simulink model "gm_DUALportRAMinterface_v3"  (R2024a)
settings: Solver=FixedStepDiscrete  StartTime=0.0  StopTime=20  RelTol=1e-3
undefined symbols (not defined in the file or in its folder): magnitude, Ts
libraries: hdlsllib x226, hdlmdlgenlib x102, embmathops x6, simulink x1, dsphdlxfrm2 x1
(part 2 of 6)

== system gm_DUALportRAMinterface_v3/PL/integration_block1/FIFO_system1 ==
  data_in : Inport  OutDataTypeStr=fixdt(1, 16, 14)  PortDimensions=1  SampleTime=3.00000003e-08
  enable_output : Inport  Port=2  OutDataTypeStr=boolean  PortDimensions=1  SampleTime=3.00000003e-08
  load_fifo : Inport  Port=3  OutDataTypeStr=boolean  PortDimensions=1  SampleTime=3.00000003e-08
  Add1 : Sum  OutDataTypeStr=fixdt(0,13,0)
  Chart1 : Subsystem
  Chart2 : Subsystem
  Chart3 : Subsystem
  Constant3 : Constant  OutDataTypeStr=fixdt(0,12,0)  SampleTime=Ts
  Constant4 : Constant  Value=0  OutDataTypeStr=fixdt(1,13,0)  SampleTime=Ts
  Delay : Delay  DelayLength=2048  InitialCondition=0  UseCircularBuffer=on
  Delay1 : Delay  DelayLength=1  InitialCondition=0  SampleTime=Ts
  Delay2 : Delay  DelayLength=1  InitialCondition=0  SampleTime=Ts
  Delay3 : Delay  DelayLength=1  InitialCondition=0
  HDL FIFO1 : hdlsllib/HDL RAMs/HDL FIFO  fifo_size=4096+2048+1  mode=Classic  ratio=1  push_msg=Warning  pop_msg=Warning  show_empty=off  show_full=on  show_num=off  LabelModeActiveChoice_Mode=Classic  rst_port=off
  Logical Operator : Logic  Operator=OR  IconShape=distinctive  AllPortsSameDT=off  OutDataTypeStr=boolean
  Logical Operator1 : Logic  IconShape=distinctive  AllPortsSameDT=off  OutDataTypeStr=boolean
  Logical Operator2 : Logic  IconShape=distinctive  AllPortsSameDT=off  OutDataTypeStr=boolean
  Logical Operator3 : Logic  Operator=XOR  IconShape=distinctive  AllPortsSameDT=off  OutDataTypeStr=boolean
  Logical Operator4 : Logic  IconShape=distinctive  AllPortsSameDT=off  OutDataTypeStr=boolean
  Logical Operator5 : Logic  Operator=XOR  IconShape=distinctive  AllPortsSameDT=off  OutDataTypeStr=boolean
  Logical Operator6 : Logic  Operator=XOR  IconShape=distinctive  AllPortsSameDT=off  OutDataTypeStr=boolean
  Switch1 : Switch  Criteria=u2 ~= 0  OutDataTypeStr=fixdt(0,13,0)  SaturateOnIntegerOverflow=off  InputSameDT=off
  Switch3 : Switch  Criteria=u2 ~= 0  OutDataTypeStr=fixdt(1, 16, 14)  SaturateOnIntegerOverflow=off  InputSameDT=off
  tuneback : Delay  DelayLength=2048+4096+0  InitialCondition=0  UseCircularBuffer=on
  data_out : Outport  SampleTime=3.00000003e-08
  data_valid : Outport  Port=2  SampleTime=3.00000003e-08
  reset_fft : Outport  Port=3  SampleTime=3.00000003e-08
  FIFO_full : Outport  Port=4  SampleTime=3.00000003e-08
  wires:
  data_in/1 -> Switch3/1
  load_fifo/1 -> Chart2/1(load_FIFO1)
  Chart3/1(enable_pop) -> Logical Operator1/1, Delay2/1, Logical Operator/2, HDL FIFO1/3
  Delay/1 -> Logical Operator2/2
  Delay2/1 -> Logical Operator1/2
  Delay3/1 -> Logical Operator6/2
  HDL FIFO1/1 -> data_out/1, Switch3/3
  HDL FIFO1/2 -> Logical Operator6/1, Delay3/1, Chart2/2(full)
  Logical Operator1/1 -> Logical Operator4/1, Logical Operator3/2, Logical Operator2/1, tuneback/1, Delay/1
  Logical Operator2/1 -> Logical Operator5/1, Logical Operator3/1
  Logical Operator3/1 -> reset_fft/1
  Logical Operator4/1 -> Logical Operator5/2
  Logical Operator5/1 -> data_valid/1
  Logical Operator6/1 -> FIFO_full/1
  Switch1/1 -> Chart3/1(counter), Delay1/1
  tuneback/1 -> Logical Operator4/2
  Logical Operator/1 -> HDL FIFO1/2
  Chart2/1(enable_push) -> Switch3/2, Logical Operator/1
  Switch3/1 -> HDL FIFO1/1
  Delay1/1 -> Chart1/1(counter), Add1/1
  enable_output/1 -> Chart1/2(en_out)
  Constant4/1 -> Switch1/3
  Constant3/1 -> Add1/2
  Chart1/1(enable_counter) -> Switch1/2
  Add1/1 -> Switch1/1

== system gm_DUALportRAMinterface_v3/PL/integration_block1/FIFO_system3 ==
  data_in : Inport  OutDataTypeStr=fixdt(1, 16, 14)  PortDimensions=1  SampleTime=3.00000003e-08
  enable_output : Inport  Port=2  OutDataTypeStr=boolean  PortDimensions=1  SampleTime=3.00000003e-08
  load_fifo : Inport  Port=3  OutDataTypeStr=boolean  PortDimensions=1  SampleTime=3.00000003e-08
  Add1 : Sum  OutDataTypeStr=fixdt(0,13,0)
  Chart1 : Subsystem
  Chart2 : Subsystem
  Chart3 : Subsystem
  Constant3 : Constant  OutDataTypeStr=fixdt(0,12,0)  SampleTime=Ts
  Constant4 : Constant  Value=0  OutDataTypeStr=fixdt(1,13,0)  SampleTime=Ts
  Delay1 : Delay  DelayLength=1  InitialCondition=0  SampleTime=Ts
  Delay3 : Delay  DelayLength=1  InitialCondition=0
  HDL FIFO1 : hdlsllib/HDL RAMs/HDL FIFO  fifo_size=4096+2048+1  mode=Classic  ratio=1  push_msg=Warning  pop_msg=Warning  show_empty=off  show_full=on  show_num=off  LabelModeActiveChoice_Mode=Classic  rst_port=off
  Logical Operator : Logic  Operator=OR  IconShape=distinctive  AllPortsSameDT=off  OutDataTypeStr=boolean
  Logical Operator6 : Logic  Operator=XOR  IconShape=distinctive  AllPortsSameDT=off  OutDataTypeStr=boolean
  Switch1 : Switch  Criteria=u2 ~= 0  OutDataTypeStr=fixdt(0,13,0)  SaturateOnIntegerOverflow=off  InputSameDT=off
  Switch3 : Switch  Criteria=u2 ~= 0  OutDataTypeStr=fixdt(1, 16, 14)  SaturateOnIntegerOverflow=off  InputSameDT=off
  t : Constant  Value=double(0)  OutDataTypeStr=boolean  SampleTime=3.00000003e-08
  t1 : Constant  Value=double(0)  OutDataTypeStr=boolean  SampleTime=3.00000003e-08
  data_out : Outport  SampleTime=3.00000003e-08
  data_valid : Outport  Port=2  SampleTime=3.00000003e-08
  reset_fft : Outport  Port=3  SampleTime=3.00000003e-08
  FIFO_full : Outport  Port=4  SampleTime=3.00000003e-08
  wires:
  data_in/1 -> Switch3/1
  load_fifo/1 -> Chart2/1(load_FIFO1)
  Chart3/1(enable_pop) -> Logical Operator/2, HDL FIFO1/3
  Delay3/1 -> Logical Operator6/2
  HDL FIFO1/1 -> data_out/1, Switch3/3
  HDL FIFO1/2 -> Logical Operator6/1, Delay3/1, Chart2/2(full)
  t1/1 -> reset_fft/1
  t/1 -> data_valid/1
  Logical Operator6/1 -> FIFO_full/1
  Switch1/1 -> Chart3/1(counter), Delay1/1
  Logical Operator/1 -> HDL FIFO1/2
  Chart2/1(enable_push) -> Switch3/2, Logical Operator/1
  Switch3/1 -> HDL FIFO1/1
  Delay1/1 -> Chart1/1(counter), Add1/1
  enable_output/1 -> Chart1/2(en_out)
  Constant4/1 -> Switch1/3
  Constant3/1 -> Add1/2
  Chart1/1(enable_counter) -> Switch1/2
  Add1/1 -> Switch1/1

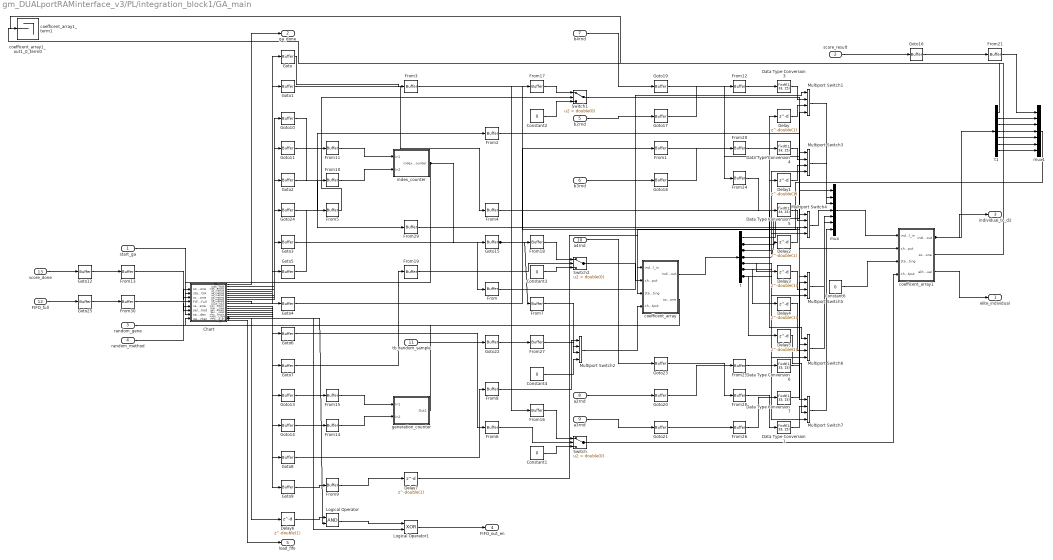
== system gm_DUALportRAMinterface_v3/PL/integration_block1/GA_main ==
  start_ga : Inport  OutDataTypeStr=boolean  PortDimensions=1  SampleTime=3.00000003e-08
  score_result : Inport  Port=2  OutDataTypeStr=fixdt(1, 33, 15)  PortDimensions=1  SampleTime=3.00000003e-08
  random_gene : Inport  Port=3  OutDataTypeStr=fixdt(0, 3, 0)  PortDimensions=1  SampleTime=3.00000003e-08
  random_method : Inport  Port=4  OutDataTypeStr=fixdt(0, 3, 0)  PortDimensions=1  SampleTime=3.00000003e-08
  b2rnd : Inport  Port=5  OutDataTypeStr=fixdt(1, 18, 15)  PortDimensions=1  SampleTime=3.00000003e-08
  b3rnd : Inport  Port=6  OutDataTypeStr=fixdt(1, 18, 15)  PortDimensions=1  SampleTime=3.00000003e-08
  b4rnd : Inport  Port=7  OutDataTypeStr=fixdt(1, 18, 15)  PortDimensions=1  SampleTime=3.00000003e-08
  a2rnd : Inport  Port=8  OutDataTypeStr=fixdt(1, 18, 15)  PortDimensions=1  SampleTime=3.00000003e-08
  a3rnd : Inport  Port=9  OutDataTypeStr=fixdt(1, 18, 15)  PortDimensions=1  SampleTime=3.00000003e-08
  a4rnd : Inport  Port=10  OutDataTypeStr=fixdt(1, 18, 15)  PortDimensions=1  SampleTime=3.00000003e-08
  tb_random_sample : Inport  Port=11  OutDataTypeStr=fixdt(0, 4, 0)  PortDimensions=1  SampleTime=3.00000003e-08
  FIFO_full : Inport  Port=12  OutDataTypeStr=boolean  PortDimensions=1  SampleTime=3.00000003e-08
  score_done : Inport  Port=13  OutDataTypeStr=boolean  PortDimensions=1  SampleTime=3.00000003e-08
  Chart : Subsystem
  Constant{1..4} (4 alike) : Constant  Value=0  OutDataTypeStr=fixdt(0, 4, 0)  SampleTime=3.00000003e-08
  Constant6 : Constant  Value=0  OutDataTypeStr=boolean  SampleTime=3.00000003e-08
  Data Type Conversion{1,3..7} (6 alike) : DataTypeConversion  OutDataTypeStr=fixdt(1, 33, 15)  SampleTime=3.00000003e-08  SaturateOnIntegerOverflow=off  RndMeth=Floor
  Delay{,1..7} (8 alike) : Delay  DelayLength=double(1)  InitialCondition=0  SampleTime=3.00000003e-08
  From{,1..21,24..30} (29 alike) : hdlmdlgenlib/Buffer
  Goto{,1..25} (26 alike) : hdlmdlgenlib/Buffer
  Logical Operator : Logic  AllPortsSameDT=off  OutDataTypeStr=boolean  SampleTime=3.00000003e-08
  Logical Operator1 : Logic  Operator=XOR  AllPortsSameDT=off  OutDataTypeStr=boolean  SampleTime=3.00000003e-08
  Multiport Switch{1,3..7} (6 alike) : MultiPortSwitch  DiagnosticForDefault=None  OutDataTypeStr=fixdt(1, 33, 15)  SampleTime=3.00000003e-08  SaturateOnIntegerOverflow=off  InputSameDT=off
  Multiport Switch2 : MultiPortSwitch  DiagnosticForDefault=None  OutDataTypeStr=fixdt(0, 4, 0)  SampleTime=3.00000003e-08  SaturateOnIntegerOverflow=off  InputSameDT=off
  Switch : Switch  Criteria=u2 > Threshold  Threshold=double(0)  OutDataTypeStr=fixdt(0, 4, 0)  SampleTime=3.00000003e-08  SaturateOnIntegerOverflow=off  InputSameDT=off
  Switch1 : Switch  Criteria=u2 > Threshold  Threshold=double(0)  OutDataTypeStr=fixdt(0, 4, 0)  SampleTime=3.00000003e-08  SaturateOnIntegerOverflow=off  InputSameDT=off
  Switch2 : Switch  Criteria=u2 > Threshold  Threshold=double(0)  OutDataTypeStr=fixdt(0, 4, 0)  SampleTime=3.00000003e-08  SaturateOnIntegerOverflow=off  InputSameDT=off
  coefficent_array : Subsystem
  coefficent_array1 : Subsystem
  coefficent_array1_out1_0_term0 : Terminator
  coefficent_array1_term1 : Terminator
  generation_counter : Subsystem
  index_counter : Subsystem
  mux : Mux  Inputs=7
  mux1 : Mux  Inputs=7
  t : Demux  Outputs=7
  t1 : Demux  Outputs=7
  elite_individual : Outport  OutDataTypeStr=fixdt(1,33,15)  SampleTime=3.00000003e-08
  ga_done : Outport  Port=2  OutDataTypeStr=boolean  SampleTime=3.00000003e-08
  individual_to_d2 : Outport  Port=3  SampleTime=3.00000003e-08
  FIFO_out_en : Outport  Port=4  SampleTime=3.00000003e-08
  load_fifo : Outport  Port=5  SampleTime=3.00000003e-08
  wires:
  score_result/1 -> Goto16/1
  b2rnd/1 -> Goto17/1
  b3rnd/1 -> Goto18/1
  b4rnd/1 -> Goto19/1
  a2rnd/1 -> Goto20/1
  a3rnd/1 -> Goto21/1
  a4rnd/1 -> Goto23/1
  tb_random_sample/1 -> Goto22/1
  FIFO_full/1 -> Goto25/1
  score_done/1 -> Goto12/1
  Chart/1(GA_done) -> ga_done/1
  Chart/17(FIFO_out_en) -> Logical Operator1/2, Logical Operator/2, Delay6/1
  Chart/18(load_fifo) -> load_fifo/1
  Delay6/1 -> Logical Operator/1
  From12/1 -> Data Type Conversion3/1
  From20/1 -> Data Type Conversion4/1
  From24/1 -> Data Type Conversion5/1
  From25/1 -> Data Type Conversion6/1
  From26/1 -> Data Type Conversion7/1
  From28/1 -> Data Type Conversion1/1
  Logical Operator/1 -> Logical Operator1/1
  Logical Operator1/1 -> FIFO_out_en/1
  coefficent_array1/1(individual_out) -> individual_to_d2/1, t1/1
  coefficent_array1/3(elite_individual) -> elite_individual/1
  Goto17/1 -> From12/1
  Goto12/1 -> From13/1
  Goto18/1 -> From20/1
  Goto16/1 -> From21/1
  Goto19/1 -> From24/1
  Goto20/1 -> From25/1
  Goto21/1 -> From26/1
  Goto22/1 -> From27/1
  Goto23/1 -> From28/1
  Goto25/1 -> From30/1
  coefficent_array1/2(sort_done) -> coefficent_array1_term1/1
  t1/1 -> coefficent_array1_out1_0_term0/1
  t1/2 -> mux1/2
  generation_counter/1(Out1) -> Chart/8(generation_counter)
  coefficent_array/1(individual_out) -> t/1
  Delay7/1 -> coefficent_array/3(start_sorting)
  index_counter/1(index_counter) -> Chart/7(sample_index), Goto15/1
  Delay/1 -> Multiport Switch1/3
  Delay1/1 -> Multiport Switch3/3
  Delay2/1 -> Multiport Switch4/3
  Delay3/1 -> Multiport Switch5/3
  Delay4/1 -> Multiport Switch6/3
  Delay5/1 -> Multiport Switch7/3
  Constant6/1 -> coefficent_array1/3(start_sorting)
  From27/1 -> Multiport Switch2/3
  Constant4/1 -> Multiport Switch2/4
  Constant3/1 -> Switch2/3
  Constant1/1 -> Switch/3
  Constant2/1 -> Switch1/3
  Data Type Conversion1/1 -> Multiport Switch7/2
  Data Type Conversion7/1 -> Multiport Switch6/2
  Data Type Conversion6/1 -> Multiport Switch5/2
  Data Type Conversion5/1 -> Multiport Switch4/2
  Data Type Conversion4/1 -> Multiport Switch3/2
  Data Type Conversion3/1 -> Multiport Switch1/2
  start_ga/1 -> Chart/2(start_GA)
  From13/1 -> Chart/3(score_done)
  From30/1 -> Chart/4(FIFO_full)
  random_gene/1 -> Chart/5(random_gene)
  random_method/1 -> Chart/6(selected_method)
  t1/3 -> mux1/3
  t1/4 -> mux1/4
  t1/5 -> mux1/5
  t1/6 -> mux1/6
  t1/7 -> mux1/7
  mux1/1 -> coefficent_array/1(individual_in)
  From21/1 -> mux1/1
  From14/1 -> generation_counter/2(In2)
  From15/1 -> generation_counter/1(In1)
  Multiport Switch2/1 -> coefficent_array/4(chose_output)
  From9/1 -> Delay7/1
  Switch2/1 -> coefficent_array/2(chose_input)
  Switch/1 -> coefficent_array1/4(chose_output)
  From10/1 -> index_counter/2(In2)
  From11/1 -> index_counter/1(In1)
  Switch1/1 -> coefficent_array1/2(chose_input)
  t/2 -> Delay/1, Multiport Switch1/4
  t/3 -> Delay1/1, Multiport Switch3/4
  t/4 -> Delay2/1, Multiport Switch4/4
  t/5 -> Delay3/1, Multiport Switch5/4
  t/6 -> Delay4/1, Multiport Switch6/4
  t/7 -> Delay5/1, Multiport Switch7/4
  mux/1 -> coefficent_array1/1(individual_in)
  coefficent_array/2(sort_done) -> Chart/1(sort_done)
  Goto14/1 -> From14/1
  Goto13/1 -> From15/1
  From7/1 -> Multiport Switch2/2
  Goto8/1 -> From8/1
  From8/1 -> Multiport Switch2/1
  Goto9/1 -> From9/1
  Goto7/1 -> From19/1
  From19/1 -> Switch2/2
  From18/1 -> Switch2/1
  Goto6/1 -> From6/1
  From6/1 -> Switch/2
  From16/1 -> Switch/1
  Goto5/1 -> From5/1
  From5/1 -> Switch1/2
  Goto10/1 -> From10/1
  Goto11/1 -> From11/1
  Goto15/1 -> From7/1, From18/1, From17/1, From16/1
  From17/1 -> Switch1/1
  Goto2/1 -> From29/1
  From29/1 -> Multiport Switch7/1
  Multiport Switch7/1 -> mux/7
  Goto1/1 -> From4/1
  From4/1 -> Multiport Switch6/1
  Multiport Switch6/1 -> mux/6
  Goto/1 -> From3/1
  From3/1 -> Multiport Switch5/1
  Multiport Switch5/1 -> mux/5
  Goto24/1 -> From2/1
  From2/1 -> Multiport Switch4/1
  Multiport Switch4/1 -> mux/4
  Goto4/1 -> From1/1
  From1/1 -> Multiport Switch3/1
  Multiport Switch3/1 -> mux/3
  Goto3/1 -> From/1
  From/1 -> Multiport Switch1/1
  Multiport Switch1/1 -> mux/2
  t/1 -> mux/1
  Chart/2(index_reset) -> Goto10/1
  Chart/3(index_increment) -> Goto11/1
  Chart/4(a2_method) -> Goto/1
  Chart/5(a3_method) -> Goto1/1
  Chart/6(a4_method) -> Goto2/1
  Chart/7(b4_method) -> Goto24/1
  Chart/8(b2_method) -> Goto3/1
  Chart/9(b3_method) -> Goto4/1
  Chart/10(slave_input) -> Goto5/1
  Chart/11(slave_output) -> Goto6/1
  Chart/12(master_input) -> Goto7/1
  Chart/13(generation_increment) -> Goto13/1
  Chart/14(generation_reset) -> Goto14/1
  Chart/15(master_output) -> Goto8/1
  Chart/16(master_sort) -> Goto9/1

== system gm_DUALportRAMinterface_v3/PL/integration_block1/Subsystem ==
  enable : Inport  OutDataTypeStr=boolean  PortDimensions=1  SampleTime=3.00000003e-08
  16bLFSR : Subsystem
  16bLFSR1 : Subsystem
  16bLFSR1_term14 : Terminator
  16bLFSR1_term15 : Terminator
  a2_random : Subsystem
  a3_random : Subsystem
  a4_random : Subsystem
  b2_random : Subsystem
  b3_random : Subsystem
  b4_random : Subsystem
  concat : hdlsllib/Logic and Bit Operations/Bit Concat  numInputs=16
  random_gene : Subsystem
  random_method : Subsystem
  random_sample : Subsystem
  random_gene_out : Outport  SampleTime=3.00000003e-08
  random_method_out : Outport  Port=2  SampleTime=3.00000003e-08
  b2_random_out : Outport  Port=3  SampleTime=3.00000003e-08
  b3_random_out : Outport  Port=4  SampleTime=3.00000003e-08
  b4_random_out : Outport  Port=5  SampleTime=3.00000003e-08
  a2_random_out : Outport  Port=6  SampleTime=3.00000003e-08
  a3_random_out : Outport  Port=7  SampleTime=3.00000003e-08
  a4_random_out : Outport  Port=8  SampleTime=3.00000003e-08
  random_sample_out : Outport  Port=9  SampleTime=3.00000003e-08
  wires:
  enable/1 -> 16bLFSR1/1(In1), 16bLFSR/1(In1)
  16bLFSR/1(y_port) -> concat/1
  16bLFSR/2(y1) -> concat/2
  16bLFSR/3(y2) -> concat/3
  16bLFSR/4(y3) -> concat/4
  16bLFSR/5(y4) -> concat/5
  16bLFSR/6(y5) -> concat/6
  16bLFSR/7(y6) -> concat/7
  16bLFSR/8(y7) -> concat/8
  16bLFSR/9(y8) -> concat/9
  16bLFSR/10(y9) -> concat/10
  16bLFSR/11(y10) -> concat/11
  16bLFSR/12(y11) -> concat/12
  16bLFSR/13(y12) -> concat/13
  16bLFSR/14(y13) -> concat/14
  16bLFSR/15(y14) -> concat/15
  16bLFSR/16(y15) -> concat/16
  16bLFSR1/1(y_port) -> a2_random/2(In2)
  16bLFSR1/2(y1) -> a3_random/2(In2)
  16bLFSR1/3(y2) -> a4_random/2(In2)
  16bLFSR1/4(y3) -> b2_random/2(In2)
  16bLFSR1/5(y4) -> b4_random/2(In2)
  16bLFSR1/6(y5) -> random_sample/1(u1)
  16bLFSR1/7(y6) -> random_sample/2(u2)
  16bLFSR1/8(y7) -> random_method/1(u1)
  16bLFSR1/9(y8) -> random_method/2(u2)
  16bLFSR1/10(y9) -> random_gene/1(u1)
  16bLFSR1/11(y10) -> random_gene/2(u2)
  16bLFSR1/12(y11) -> random_gene/3(In3)
  16bLFSR1/13(y12) -> b3_random/2(In2)
  16bLFSR1/14(y13) -> random_gene/4(In4)
  a2_random/1(Out1) -> a2_random_out/1
  a3_random/1(Out1) -> a3_random_out/1
  a4_random/1(Out1) -> a4_random_out/1
  b2_random/1(Out1) -> b2_random_out/1
  b3_random/1(Out1) -> b3_random_out/1
  b4_random/1(Out1) -> b4_random_out/1
  concat/1 -> a3_random/1(In1), a2_random/1(In1), b3_random/1(In1), b2_random/1(In1), b4_random/1(In1), a4_random/1(In1)
  random_gene/1(Out1) -> random_gene_out/1
  random_method/1(Out1) -> random_method_out/1
  random_sample/1(Out1) -> random_sample_out/1
  16bLFSR1/15(y14) -> 16bLFSR1_term14/1
  16bLFSR1/16(y15) -> 16bLFSR1_term15/1

== system gm_DUALportRAMinterface_v3/PL/integration_block1/accumulator_scorer ==
  data_in : Inport  OutDataTypeStr=fixdt(1, 28, 14)  PortDimensions=1  SampleTime=3.00000003e-08
      settings: SignalType=complex
  valid_fft : Inport  Port=2  OutDataTypeStr=boolean  PortDimensions=1  SampleTime=3.00000003e-08
  64bitmsb_finder : Subsystem
  Add : Sum  OutDataTypeStr=fixdt(1,64,32)  AccumDataTypeStr=fixdt(1,64,32)  SaturateOnIntegerOverflow=on
  Add2 : Sum  OutDataTypeStr=fixdt(1, 64, 32)  AccumDataTypeStr=fixdt(1,64,32)  SaturateOnIntegerOverflow=on
  Complex to Real-Imag : ComplexToRealImag
  Constant1 : Constant  Value=0  OutDataTypeStr=fixdt(1,26,12)  SampleTime=Ts
  Constant19 : Constant  Value=0  OutDataTypeStr=fixdt(1,26,12)  SampleTime=Ts
  Constant20 : Constant  Value=0  OutDataTypeStr=fixdt(1,64,32)  SampleTime=Ts
  Data Type Conversion : DataTypeConversion  OutDataTypeStr=fixdt(1,64,32)  SaturateOnIntegerOverflow=off  RndMeth=Floor
  Data Type Conversion1 : DataTypeConversion  OutDataTypeStr=fixdt(1,64,32)  SaturateOnIntegerOverflow=off  RndMeth=Floor
  Data Type Conversion2 : DataTypeConversion  OutDataTypeStr=fixdt(1,33,15)  SaturateOnIntegerOverflow=off  RndMeth=Floor
  Delay : Delay  DelayLength=1  InitialCondition=0  SampleTime=Ts
  Delay1 : Delay  DelayLength=63  InitialCondition=0
  Delay2 : Delay  DelayLength=1  InitialCondition=0
  Delay3 : Delay  DelayLength=4096-64  InitialCondition=0  UseCircularBuffer=on
  Logical Operator1 : Logic  IconShape=distinctive  AllPortsSameDT=off  OutDataTypeStr=boolean
  Logical Operator2 : Logic  IconShape=distinctive  AllPortsSameDT=off  OutDataTypeStr=boolean
  Magnitude Square1 : Math  Operator=magnitude^2  SignedPower=on  OutputSignalType=real  OutDataTypeStr=fixdt(1, 64, 32)  RndMeth=Zero
  Magnitude Square2 : Math  Operator=magnitude^2  SignedPower=on  OutputSignalType=real  OutDataTypeStr=fixdt(1, 64, 32)  RndMeth=Zero
  Real-Imag to Complex : RealImagToComplex
  Switch : Switch  Criteria=u2 > Threshold  OutDataTypeStr=fixdt(1, 28, 14)  SaturateOnIntegerOverflow=off  InputSameDT=off
  Switch8 : Switch  Criteria=u2 > Threshold  OutDataTypeStr=fixdt(1,64,32)  InputSameDT=off
  individual_score : Outport  SampleTime=3.00000003e-08
  individual_score_valid : Outport  Port=2  SampleTime=3.00000003e-08
  wires:
  data_in/1 -> Switch/1
  valid_fft/1 -> Logical Operator1/1, Delay3/1
  Add2/1 -> 64bitmsb_finder/1(u_port)
  Complex to Real-Imag/1 -> Data Type Conversion/1
  Complex to Real-Imag/2 -> Data Type Conversion1/1
  Constant1/1 -> Real-Imag to Complex/2
  Constant19/1 -> Real-Imag to Complex/1
  Data Type Conversion/1 -> Magnitude Square1/1
  Data Type Conversion1/1 -> Magnitude Square2/1
  Data Type Conversion2/1 -> individual_score/1
  Delay/1 -> Data Type Conversion2/1, Switch8/1
  Delay1/1 -> Logical Operator2/1
  Delay2/1 -> individual_score_valid/1
  Delay3/1 -> Logical Operator1/2
  Logical Operator1/1 -> Switch/2, Logical Operator2/2, [reset_lol], Delay1/1
  Logical Operator2/1 -> Delay2/1
  Magnitude Square1/1 -> Add2/1
  Magnitude Square2/1 -> Add2/2
  Real-Imag to Complex/1 -> Switch/3
  Switch/1 -> Complex to Real-Imag/1
  [reset_lol] -> Switch8/2
  Constant20/1 -> Switch8/3
  64bitmsb_finder/1(out1) -> Add/1
  Add/1 -> Delay/1
  Switch8/1 -> Add/2

== system gm_DUALportRAMinterface_v3/PL/integration_block1/D2/individual1 ==
  reg_in : Inport  OutDataTypeStr=fixdt(1, 33, 15)  PortDimensions=1  SampleTime=3.00000003e-08
  reg_in1 : Inport  Port=2  OutDataTypeStr=fixdt(1, 33, 15)  PortDimensions=1  SampleTime=3.00000003e-08
  reg_in2 : Inport  Port=3  OutDataTypeStr=fixdt(1, 33, 15)  PortDimensions=1  SampleTime=3.00000003e-08
  reg_in3 : Inport  Port=4  OutDataTypeStr=fixdt(1, 33, 15)  PortDimensions=1  SampleTime=3.00000003e-08
  reg_in4 : Inport  Port=5  OutDataTypeStr=fixdt(1, 33, 15)  PortDimensions=1  SampleTime=3.00000003e-08
  reg_in5 : Inport  Port=6  OutDataTypeStr=fixdt(1, 33, 15)  PortDimensions=1  SampleTime=3.00000003e-08
  reg_in6 : Inport  Port=7  OutDataTypeStr=fixdt(1, 33, 15)  PortDimensions=1  SampleTime=3.00000003e-08
  enable : Inport  Port=8  OutDataTypeStr=boolean  PortDimensions=1  SampleTime=3.00000003e-08
  Subsystem1 : Subsystem
  Subsystem2 : Subsystem
  Subsystem3 : Subsystem
  Subsystem4 : Subsystem
  Subsystem5 : Subsystem
  Subsystem6 : Subsystem
  reg_in_term0 : Terminator
  t : Constant  Value=fi(0,1,33,15)  OutDataTypeStr=fixdt(1, 33, 15)  SampleTime=3.00000003e-08
  score : Outport  SampleTime=3.00000003e-08
  a2 : Outport  Port=2  SampleTime=3.00000003e-08
  a3 : Outport  Port=3  SampleTime=3.00000003e-08
  a4 : Outport  Port=4  SampleTime=3.00000003e-08
  b2 : Outport  Port=5  SampleTime=3.00000003e-08
  b3 : Outport  Port=6  SampleTime=3.00000003e-08
  b4 : Outport  Port=7  SampleTime=3.00000003e-08
  wires:
  reg_in/1 -> reg_in_term0/1
  reg_in1/1 -> Subsystem1/1(reg_in)
  reg_in2/1 -> Subsystem2/1(reg_in)
  reg_in3/1 -> Subsystem3/1(reg_in)
  reg_in4/1 -> Subsystem4/1(reg_in)
  reg_in5/1 -> Subsystem5/1(reg_in)
  reg_in6/1 -> Subsystem6/1(reg_in)
  enable/1 -> Subsystem3/2(enable), Subsystem4/2(enable), Subsystem5/2(enable), Subsystem6/2(enable), Subsystem2/2(enable), Subsystem1/2(enable)
  t/1 -> score/1
  Subsystem1/1(reg_out) -> a2/1
  Subsystem2/1(reg_out) -> a3/1
  Subsystem3/1(reg_out) -> a4/1
  Subsystem4/1(reg_out) -> b2/1
  Subsystem5/1(reg_out) -> b3/1
  Subsystem6/1(reg_out) -> b4/1

== system gm_DUALportRAMinterface_v3/PL/integration_block1/D2/output_cast1 ==
  in : Inport  OutDataTypeStr=fixdt(1, 14, 12)  SampleTime=3.00000003e-08
  out : Outport  SampleTime=3.00000003e-08
  wires:
  in/1 -> out/1

== system gm_DUALportRAMinterface_v3/PL/integration_block1/FIFO_system1/Chart1 ==
  counter : Inport  OutDataTypeStr=fixdt(0, 13, 0)  PortDimensions=1  SampleTime=3.00000003e-08
  en_out : Inport  Port=2  OutDataTypeStr=boolean  PortDimensions=1  SampleTime=3.00000003e-08
  Chart1 : Stateflow chart  TreatAsAtomicUnit=on
      settings: PortSchema="{\"entries\":[{\"content\":{\"sides\":[{\"content\":{\"connectorIds\":[\"In2\"]},\"type\":\"ConnectorPlacement.EquallySpacedRectSide\",\"uuid\":\"9d6f18ef-7bce-40b0-94a2-758e33355834\"},{\"content\":{\"connectorIds\":[\"Out1\"],\"side\":\"RIGHT\"},\"type\":\"ConnectorPlacement.EquallySpacedRectSide\",\"uuid\":\"7bab70ba-8111-4145-9c29-33f98ce79820\"},{\"content\":{\"side\":\"TOP\"},\"type\":\"ConnectorPlacement.EquallySpacedRectSide\",\"uuid\":\"d3288235-814f-4c71-bec2-04d07c53d63c\"},{\"content\":{\"connectorIds\":[\"In1\"],\"side\":\"BOTTOM\"},\"type\":\"ConnectorPlacement.EquallySpacedRectSide\",\"uuid\":\"018953e5-55f4-4114-8f5d-132f3f7565f7\"}]},\"type\":\"ConnectorPlacement.EquallySpacedConnector\",\"uuid\":\"70011da9-c6ae-4e69-953f-1d8cbe8c7c12\"}],\"packageUris\":[\"http://schema.mathworks.com/mf0/Connector/R2020b\"],\"version\":\"1.0\"}"
  enable_counter : Outport  SampleTime=3.00000003e-08
  wires:
  Chart1/1(enable_counter) -> enable_counter/1
  en_out/1 -> Chart1/2(en_out)
  counter/1 -> Chart1/1(counter)

== system gm_DUALportRAMinterface_v3/PL/integration_block1/FIFO_system1/Chart2 ==
  load_FIFO1 : Inport  OutDataTypeStr=boolean  PortDimensions=1  SampleTime=3.00000003e-08
  full : Inport  Port=2  OutDataTypeStr=boolean  PortDimensions=1  SampleTime=3.00000003e-08
  Chart2 : Stateflow chart  TreatAsAtomicUnit=on
      settings: PortSchema="{\"entries\":[{\"content\":{\"sides\":[{\"content\":{\"connectorIds\":[\"In1\"]},\"type\":\"ConnectorPlacement.EquallySpacedRectSide\",\"uuid\":\"9d6f18ef-7bce-40b0-94a2-758e33355834\"},{\"content\":{\"connectorIds\":[\"Out1\"],\"side\":\"RIGHT\"},\"type\":\"ConnectorPlacement.EquallySpacedRectSide\",\"uuid\":\"7bab70ba-8111-4145-9c29-33f98ce79820\"},{\"content\":{\"connectorIds\":[\"In2\"],\"side\":\"TOP\"},\"type\":\"ConnectorPlacement.EquallySpacedRectSide\",\"uuid\":\"d3288235-814f-4c71-bec2-04d07c53d63c\"}]},\"type\":\"ConnectorPlacement.EquallySpacedConnector\",\"uuid\":\"70011da9-c6ae-4e69-953f-1d8cbe8c7c12\"}],\"packageUris\":[\"http://schema.mathworks.com/mf0/Connector/R2020b\"],\"version\":\"1.0\"}"
  enable_push : Outport  SampleTime=3.00000003e-08
  wires:
  Chart2/1(enable_push) -> enable_push/1
  full/1 -> Chart2/2(full)
  load_FIFO1/1 -> Chart2/1(load_FIFO1)

== system gm_DUALportRAMinterface_v3/PL/integration_block1/FIFO_system1/Chart3 ==
  counter : Inport  OutDataTypeStr=fixdt(0, 13, 0)  PortDimensions=1  SampleTime=3.00000003e-08
  Chart3 : Stateflow chart  TreatAsAtomicUnit=on
  enable_pop : Outport  SampleTime=3.00000003e-08
  wires:
  Chart3/1(enable_pop) -> enable_pop/1
  counter/1 -> Chart3/1(counter)

== system gm_DUALportRAMinterface_v3/PL/integration_block1/FIFO_system3/Chart1 ==
  counter : Inport  OutDataTypeStr=fixdt(0, 13, 0)  PortDimensions=1  SampleTime=3.00000003e-08
  en_out : Inport  Port=2  OutDataTypeStr=boolean  PortDimensions=1  SampleTime=3.00000003e-08
  Chart1 : Stateflow chart  TreatAsAtomicUnit=on
      settings: PortSchema="{\"entries\":[{\"content\":{\"sides\":[{\"content\":{\"connectorIds\":[\"In2\"]},\"type\":\"ConnectorPlacement.EquallySpacedRectSide\",\"uuid\":\"9d6f18ef-7bce-40b0-94a2-758e33355834\"},{\"content\":{\"connectorIds\":[\"Out1\"],\"side\":\"RIGHT\"},\"type\":\"ConnectorPlacement.EquallySpacedRectSide\",\"uuid\":\"7bab70ba-8111-4145-9c29-33f98ce79820\"},{\"content\":{\"side\":\"TOP\"},\"type\":\"ConnectorPlacement.EquallySpacedRectSide\",\"uuid\":\"d3288235-814f-4c71-bec2-04d07c53d63c\"},{\"content\":{\"connectorIds\":[\"In1\"],\"side\":\"BOTTOM\"},\"type\":\"ConnectorPlacement.EquallySpacedRectSide\",\"uuid\":\"018953e5-55f4-4114-8f5d-132f3f7565f7\"}]},\"type\":\"ConnectorPlacement.EquallySpacedConnector\",\"uuid\":\"70011da9-c6ae-4e69-953f-1d8cbe8c7c12\"}],\"packageUris\":[\"http://schema.mathworks.com/mf0/Connector/R2020b\"],\"version\":\"1.0\"}"
  enable_counter : Outport  SampleTime=3.00000003e-08
  wires:
  counter/1 -> Chart1/1(counter)
  en_out/1 -> Chart1/2(en_out)
  Chart1/1(enable_counter) -> enable_counter/1

== system gm_DUALportRAMinterface_v3/PL/integration_block1/FIFO_system3/Chart2 ==
  load_FIFO1 : Inport  OutDataTypeStr=boolean  PortDimensions=1  SampleTime=3.00000003e-08
  full : Inport  Port=2  OutDataTypeStr=boolean  PortDimensions=1  SampleTime=3.00000003e-08
  Chart2 : Stateflow chart  TreatAsAtomicUnit=on
      settings: PortSchema="{\"entries\":[{\"content\":{\"sides\":[{\"content\":{\"connectorIds\":[\"In1\"]},\"type\":\"ConnectorPlacement.EquallySpacedRectSide\",\"uuid\":\"9d6f18ef-7bce-40b0-94a2-758e33355834\"},{\"content\":{\"connectorIds\":[\"Out1\"],\"side\":\"RIGHT\"},\"type\":\"ConnectorPlacement.EquallySpacedRectSide\",\"uuid\":\"7bab70ba-8111-4145-9c29-33f98ce79820\"},{\"content\":{\"connectorIds\":[\"In2\"],\"side\":\"TOP\"},\"type\":\"ConnectorPlacement.EquallySpacedRectSide\",\"uuid\":\"d3288235-814f-4c71-bec2-04d07c53d63c\"}]},\"type\":\"ConnectorPlacement.EquallySpacedConnector\",\"uuid\":\"70011da9-c6ae-4e69-953f-1d8cbe8c7c12\"}],\"packageUris\":[\"http://schema.mathworks.com/mf0/Connector/R2020b\"],\"version\":\"1.0\"}"
  enable_push : Outport  SampleTime=3.00000003e-08
  wires:
  load_FIFO1/1 -> Chart2/1(load_FIFO1)
  full/1 -> Chart2/2(full)
  Chart2/1(enable_push) -> enable_push/1

== system gm_DUALportRAMinterface_v3/PL/integration_block1/FIFO_system3/Chart3 ==
  counter : Inport  OutDataTypeStr=fixdt(0, 13, 0)  PortDimensions=1  SampleTime=3.00000003e-08
  Chart3 : Stateflow chart  TreatAsAtomicUnit=on
  enable_pop : Outport  SampleTime=3.00000003e-08
  wires:
  counter/1 -> Chart3/1(counter)
  Chart3/1(enable_pop) -> enable_pop/1

== system gm_DUALportRAMinterface_v3/PL/integration_block1/GA_main/Chart ==
  sort_done : Inport  OutDataTypeStr=boolean  PortDimensions=1  SampleTime=3.00000003e-08
  start_GA : Inport  Port=2  OutDataTypeStr=boolean  PortDimensions=1  SampleTime=3.00000003e-08
  score_done : Inport  Port=3  OutDataTypeStr=boolean  PortDimensions=1  SampleTime=3.00000003e-08
  FIFO_full : Inport  Port=4  OutDataTypeStr=boolean  PortDimensions=1  SampleTime=3.00000003e-08
  random_gene : Inport  Port=5  OutDataTypeStr=fixdt(0, 3, 0)  PortDimensions=1  SampleTime=3.00000003e-08
  selected_method : Inport  Port=6  OutDataTypeStr=fixdt(0, 3, 0)  PortDimensions=1  SampleTime=3.00000003e-08
  sample_index : Inport  Port=7  OutDataTypeStr=fixdt(0, 4, 0)  PortDimensions=1  SampleTime=3.00000003e-08
  generation_counter : Inport  Port=8  OutDataTypeStr=uint16  PortDimensions=1  SampleTime=3.00000003e-08
  Chart : Stateflow chart  TreatAsAtomicUnit=on
      settings: PortSchema="{\"entries\":[{\"content\":{\"sides\":[{\"content\":{\"connectorIds\":[\"In1\",\"In2\",\"In3\",\"In4\",\"In5\",\"In6\",\"In7\",\"In8\"]},\"type\":\"ConnectorPlacement.EquallySpacedRectSide\",\"uuid\":\"62d80992-ebbf-487b-a33b-520d46b16df9\"},{\"content\":{\"connectorIds\":[\"Out1\",\"Out4\",\"Out5\",\"Out6\",\"Out8\",\"Out9\",\"Out7\",\"Out10\",\"Out11\",\"Out12\",\"Out15\",\"Out16\",\"Out13\",\"Out14\",\"Out3\",\"Out2\",\"Out17\",\"Out18\"],\"side\":\"RIGHT\"},\"type\":\"ConnectorPlacement.EquallySpacedRectSide\",\"uuid\":\"bfd840c0-5c4c-4a80-a2e3-fe311b40edf5\"},{\"content\":{\"side\":\"TOP\"},\"type\":\"ConnectorPlacement.EquallySpacedRectSide\",\"uuid\":\"4ac6e66e-dbf9-46cb-9f74-339923e0521f\"},{\"content\":{\"side\":\"BOTTOM\"},\"type\":\"ConnectorPlacement.EquallySpacedRectSide\",\"uuid\":\"c9defcd3-49e4-4e79-8497-0d4d1ccc3a89\"}]},\"type\":\"ConnectorPlacement.EquallySpacedConnector\",\"uuid\":\"f0f6ce29-0824-409a-b95e-7d534cdcf216\"}],\"packageUris\":[\"http://schema.mathworks.com/mf0/Connector/R2020b\"],\"version\":\"1.0\"}"
  GA_done : Outport  SampleTime=3.00000003e-08
  index_reset : Outport  Port=2  SampleTime=3.00000003e-08
  index_increment : Outport  Port=3  SampleTime=3.00000003e-08
  a2_method : Outport  Port=4  SampleTime=3.00000003e-08
  a3_method : Outport  Port=5  SampleTime=3.00000003e-08
  a4_method : Outport  Port=6  SampleTime=3.00000003e-08
  b4_method : Outport  Port=7  SampleTime=3.00000003e-08
  b2_method : Outport  Port=8  SampleTime=3.00000003e-08
  b3_method : Outport  Port=9  SampleTime=3.00000003e-08
  slave_input : Outport  Port=10  SampleTime=3.00000003e-08
  slave_output : Outport  Port=11  SampleTime=3.00000003e-08
  master_input : Outport  Port=12  SampleTime=3.00000003e-08
  generation_increment : Outport  Port=13  SampleTime=3.00000003e-08
  generation_reset : Outport  Port=14  SampleTime=3.00000003e-08
  master_output : Outport  Port=15  SampleTime=3.00000003e-08
  master_sort : Outport  Port=16  SampleTime=3.00000003e-08
  FIFO_out_en : Outport  Port=17  SampleTime=3.00000003e-08
  load_fifo : Outport  Port=18  SampleTime=3.00000003e-08
  wires:
  sort_done/1 -> Chart/1(sort_done)
  start_GA/1 -> Chart/2(start_GA)
  score_done/1 -> Chart/3(score_done)
  FIFO_full/1 -> Chart/4(FIFO_full)
  random_gene/1 -> Chart/5(random_gene)
  selected_method/1 -> Chart/6(selected_method)
  sample_index/1 -> Chart/7(sample_index)
  generation_counter/1 -> Chart/8(generation_counter)
  Chart/1(GA_done) -> GA_done/1
  Chart/2(index_reset) -> index_reset/1
  Chart/3(index_increment) -> index_increment/1
  Chart/4(a2_method) -> a2_method/1
  Chart/5(a3_method) -> a3_method/1
  Chart/6(a4_method) -> a4_method/1
  Chart/7(b4_method) -> b4_method/1
  Chart/8(b2_method) -> b2_method/1
  Chart/9(b3_method) -> b3_method/1
  Chart/10(slave_input) -> slave_input/1
  Chart/11(slave_output) -> slave_output/1
  Chart/12(master_input) -> master_input/1
  Chart/13(generation_increment) -> generation_increment/1
  Chart/14(generation_reset) -> generation_reset/1
  Chart/15(master_output) -> master_output/1
  Chart/16(master_sort) -> master_sort/1
  Chart/17(FIFO_out_en) -> FIFO_out_en/1
  Chart/18(load_fifo) -> load_fifo/1

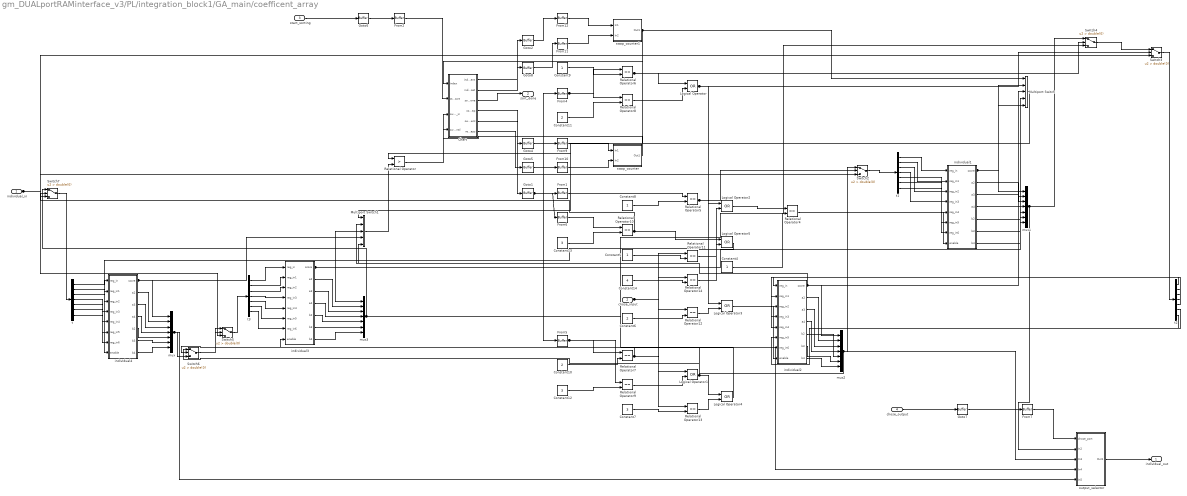
== system gm_DUALportRAMinterface_v3/PL/integration_block1/GA_main/coefficent_array ==
  individual_in : Inport  OutDataTypeStr=fixdt(1, 33, 15)  PortDimensions=[7]  SampleTime=3.00000003e-08
  chose_input : Inport  Port=2  OutDataTypeStr=fixdt(0, 4, 0)  PortDimensions=1  SampleTime=3.00000003e-08
  start_sorting : Inport  Port=3  OutDataTypeStr=boolean  PortDimensions=1  SampleTime=3.00000003e-08
  chose_output : Inport  Port=4  OutDataTypeStr=fixdt(0, 4, 0)  PortDimensions=1  SampleTime=3.00000003e-08
  Chart : Subsystem
  Constant10 : Constant  Value=2  OutDataTypeStr=fixdt(0, 4, 0)  SampleTime=3.00000003e-08
  Constant11 : Constant  Value=2  OutDataTypeStr=fixdt(0, 4, 0)  SampleTime=3.00000003e-08
  Constant12 : Constant  Value=3  OutDataTypeStr=fixdt(0, 4, 0)  SampleTime=3.00000003e-08
  Constant13 : Constant  Value=3  OutDataTypeStr=fixdt(0, 4, 0)  SampleTime=3.00000003e-08
  Constant14 : Constant  Value=4  OutDataTypeStr=fixdt(0, 4, 0)  SampleTime=3.00000003e-08
  Constant{4..5,8..9} (4 alike) : Constant  OutDataTypeStr=fixdt(0, 4, 0)  SampleTime=3.00000003e-08
  Constant6 : Constant  Value=2  OutDataTypeStr=fixdt(0, 4, 0)  SampleTime=3.00000003e-08
  Constant7 : Constant  Value=3  OutDataTypeStr=fixdt(0, 4, 0)  SampleTime=3.00000003e-08
  From{1..2,4..7,9..12} (10 alike) : hdlmdlgenlib/Buffer
  Goto{1..2,4..8} (7 alike) : hdlmdlgenlib/Buffer
  Logical Operator{,1..5} (6 alike) : Logic  Operator=OR  AllPortsSameDT=off  OutDataTypeStr=boolean  SampleTime=3.00000003e-08
  Multiport Switch : MultiPortSwitch  DataPortForDefault=Additional data port  DiagnosticForDefault=None  OutDataTypeStr=fixdt(1, 33, 15)  SampleTime=3.00000003e-08  SaturateOnIntegerOverflow=off  InputSameDT=off
  Multiport Switch1 : MultiPortSwitch  DataPortForDefault=Additional data port  DiagnosticForDefault=None  OutDataTypeStr=fixdt(1, 33, 15)  SampleTime=3.00000003e-08  SaturateOnIntegerOverflow=off  InputSameDT=off
  Relational Operator : RelationalOperator  Operator=>  OutDataTypeStr=boolean  SampleTime=3.00000003e-08  InputSameDT=off
  Relational Operator{4..14} (11 alike) : RelationalOperator  Operator===  OutDataTypeStr=boolean  SampleTime=3.00000003e-08  InputSameDT=off
  Switch{2..7} (6 alike) : Switch  Criteria=u2 > Threshold  Threshold=double(0)  OutDataTypeStr=fixdt(1, 33, 15)  SampleTime=3.00000003e-08  SaturateOnIntegerOverflow=off  InputSameDT=off
  individual1 : Subsystem
  individual2 : Subsystem
  individual3 : Subsystem
  individual4 : Subsystem
  mux{,1..3} (4 alike) : Mux  Inputs=7
  output_selector : Subsystem
  swap_counter : Subsystem
  swap_counter1 : Subsystem
  t{,1..3} (4 alike) : Demux  Outputs=7
  individual_out : Outport  SampleTime=3.00000003e-08
  sort_done : Outport  Port=2  SampleTime=3.00000003e-08
  wires:
  chose_input/1 -> Relational Operator14/1, Relational Operator13/1, Relational Operator12/1, Relational Operator11/1
  start_sorting/1 -> Goto6/1
  chose_output/1 -> Goto7/1
  Chart/3(sort_done) -> sort_done/1
  Constant14/1 -> Relational Operator14/2
  Constant5/1 -> Relational Operator11/2
  Constant6/1 -> Relational Operator12/2
  Constant7/1 -> Relational Operator13/2
  From7/1 -> output_selector/1(chose_port)
  mux1/1 -> output_selector/2(In2), Switch4/1
  mux2/1 -> output_selector/3(In3), Switch6/1, Switch2/1
  mux3/1 -> output_selector/4(In4), Switch7/1, Switch4/3
  mux/1 -> output_selector/5(In5), Switch6/3
  output_selector/1(Out1) -> individual_out/1
  Goto6/1 -> From2/1
  Goto7/1 -> From7/1
  individual3/1(score) -> Multiport Switch/4, Multiport Switch1/3, mux3/1
  individual3/2(a2) -> mux3/2
  individual3/3(a3) -> mux3/3
  individual3/4(a4) -> mux3/4
  individual3/5(b2) -> mux3/5
  individual3/6(b3) -> mux3/6
  individual3/7(b4) -> mux3/7
  individual2/1(score) -> Multiport Switch/3, Multiport Switch1/2, Multiport Switch1/5, mux2/1
  individual2/2(a2) -> mux2/2
  individual2/3(a3) -> mux2/3
  individual2/4(a4) -> mux2/4
  individual2/5(b2) -> mux2/5
  individual2/6(b3) -> mux2/6
  individual2/7(b4) -> mux2/7
  individual1/1(score) -> Multiport Switch/2, Multiport Switch/5, mux1/1
  individual1/2(a2) -> mux1/2
  individual1/3(a3) -> mux1/3
  individual1/4(a4) -> mux1/4
  individual1/5(b2) -> mux1/5
  individual1/6(b3) -> mux1/6
  individual1/7(b4) -> mux1/7
  individual4/1(score) -> Multiport Switch1/4, mux/1
  individual4/2(a2) -> mux/2
  individual4/3(a3) -> mux/3
  individual4/4(a4) -> mux/4
  individual4/5(b2) -> mux/5
  individual4/6(b3) -> mux/6
  individual4/7(b4) -> mux/7
  swap_counter/1(Out1) -> Chart/3(swaps_in)
  swap_counter1/1(Out1) -> Chart/1(index), Multiport Switch/1, Multiport Switch1/1
  Relational Operator13/1 -> Logical Operator4/2
  Constant12/1 -> Relational Operator9/2
  Constant10/1 -> Relational Operator7/2
  Relational Operator12/1 -> Logical Operator3/2
  Constant11/1 -> Relational Operator8/2
  Constant9/1 -> Relational Operator6/2
  Relational Operator11/1 -> Logical Operator2/2
  Constant4/1 -> Relational Operator4/2
  Relational Operator14/1 -> Logical Operator5/2
  Constant13/1 -> Relational Operator10/2
  individual_in/1 -> Switch7/3, Switch5/3, Switch3/3, Switch2/3
  From2/1 -> Chart/2(start_sort)
  Constant8/1 -> Relational Operator5/2
  Logical Operator4/1 -> individual3/8(enable)
  Logical Operator3/1 -> individual2/8(enable)
  Relational Operator4/1 -> individual1/8(enable)
  Logical Operator5/1 -> individual4/8(enable)
  t/1 -> individual4/1(reg_in)
  t/2 -> individual4/2(reg_in1)
  t/3 -> individual4/3(reg_in2)
  t/4 -> individual4/4(reg_in3)
  t/5 -> individual4/5(reg_in4)
  t/6 -> individual4/6(reg_in5)
  t/7 -> individual4/7(reg_in6)
  From10/1 -> swap_counter/2(In2)
  From9/1 -> swap_counter/1(In1)
  From11/1 -> swap_counter1/2(In2)
  From12/1 -> swap_counter1/1(In1)
  t1/1 -> individual1/1(reg_in)
  t1/2 -> individual1/2(reg_in1)
  t1/3 -> individual1/3(reg_in2)
  t1/4 -> individual1/4(reg_in3)
  t1/5 -> individual1/5(reg_in4)
  t1/6 -> individual1/6(reg_in5)
  t1/7 -> individual1/7(reg_in6)
  t2/1 -> individual2/1(reg_in)
  t2/2 -> individual2/2(reg_in1)
  t2/3 -> individual2/3(reg_in2)
  t2/4 -> individual2/4(reg_in3)
  t2/5 -> individual2/5(reg_in4)
  t2/6 -> individual2/6(reg_in5)
  t2/7 -> individual2/7(reg_in6)
  t3/1 -> individual3/1(reg_in)
  t3/2 -> individual3/2(reg_in1)
  t3/3 -> individual3/3(reg_in2)
  t3/4 -> individual3/4(reg_in3)
  t3/5 -> individual3/5(reg_in4)
  t3/6 -> individual3/6(reg_in5)
  t3/7 -> individual3/7(reg_in6)
  Relational Operator9/1 -> Logical Operator1/2
  Logical Operator1/1 -> Switch5/2, Logical Operator4/1
  From5/1 -> Relational Operator9/1, Relational Operator7/1
  Relational Operator7/1 -> Switch6/2, Logical Operator1/1
  Relational Operator8/1 -> Logical Operator/2
  Logical Operator/1 -> Switch3/2, Logical Operator3/1
  From4/1 -> Relational Operator8/1, Relational Operator6/1
  Relational Operator6/1 -> Switch4/2, Logical Operator/1
  Logical Operator2/1 -> Relational Operator4/1
  From6/1 -> Relational Operator10/1
  Relational Operator10/1 -> Switch7/2, Logical Operator5/1
  Switch7/1 -> t/1
  Multiport Switch1/1 -> Relational Operator/2
  Multiport Switch/1 -> Relational Operator/1
  Relational Operator/1 -> Chart/4(swap_signal)
  Goto5/1 -> From10/1
  Goto4/1 -> From9/1
  Goto8/1 -> From11/1
  Goto2/1 -> From12/1
  Chart/1(index_increment) -> Goto2/1
  Chart/2(index_reset) -> Goto8/1
  Chart/4(commit_swap) -> Goto1/1
  Chart/5(swaps_increment) -> Goto4/1
  Chart/6(reset_swaps) -> Goto5/1
  Goto1/1 -> From6/1, From5/1, From4/1, From1/1
  From1/1 -> Relational Operator5/1
  Relational Operator5/1 -> Switch2/2, Logical Operator2/1
  Switch2/1 -> t1/1
  Switch4/1 -> Switch3/1
  Switch3/1 -> t2/1
  Switch6/1 -> Switch5/1
  Switch5/1 -> t3/1

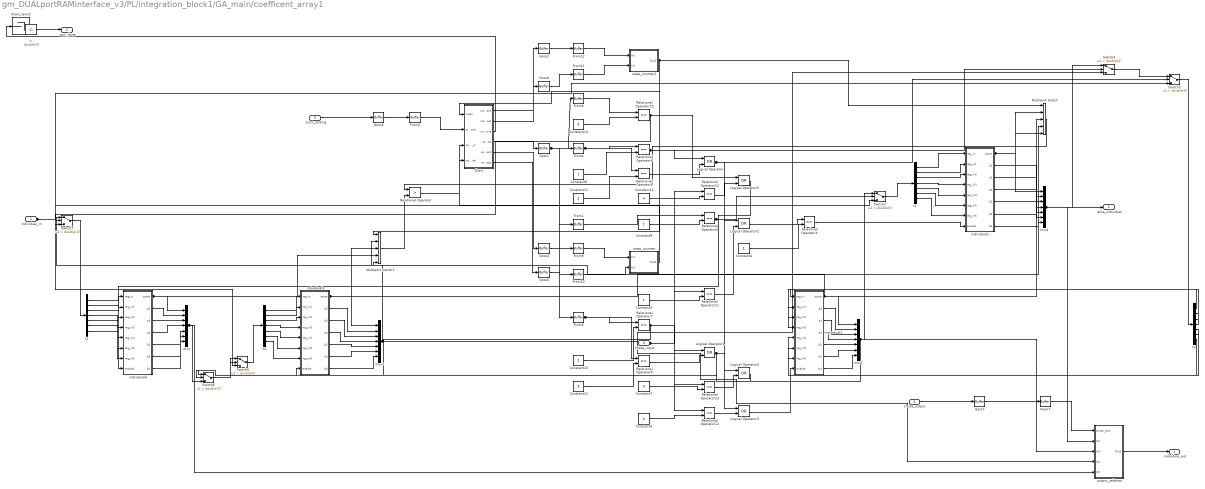
== system gm_DUALportRAMinterface_v3/PL/integration_block1/GA_main/coefficent_array1 ==
  individual_in : Inport  OutDataTypeStr=fixdt(1, 33, 15)  PortDimensions=[7]  SampleTime=3.00000003e-08
  chose_input : Inport  Port=2  OutDataTypeStr=fixdt(0, 4, 0)  PortDimensions=1  SampleTime=3.00000003e-08
  start_sorting : Inport  Port=3  OutDataTypeStr=boolean  PortDimensions=1  SampleTime=3.00000003e-08
  chose_output : Inport  Port=4  OutDataTypeStr=fixdt(0, 4, 0)  PortDimensions=1  SampleTime=3.00000003e-08
  Chart : Subsystem
  Chart_term2 : Terminator
  Constant10 : Constant  Value=2  OutDataTypeStr=fixdt(0, 4, 0)  SampleTime=3.00000003e-08
  Constant11 : Constant  Value=2  OutDataTypeStr=fixdt(0, 4, 0)  SampleTime=3.00000003e-08
  Constant12 : Constant  Value=3  OutDataTypeStr=fixdt(0, 4, 0)  SampleTime=3.00000003e-08
  Constant13 : Constant  Value=3  OutDataTypeStr=fixdt(0, 4, 0)  SampleTime=3.00000003e-08
  Constant14 : Constant  Value=4  OutDataTypeStr=fixdt(0, 4, 0)  SampleTime=3.00000003e-08
  Constant{4..5,8..9} (4 alike) : Constant  OutDataTypeStr=fixdt(0, 4, 0)  SampleTime=3.00000003e-08
  Constant6 : Constant  Value=2  OutDataTypeStr=fixdt(0, 4, 0)  SampleTime=3.00000003e-08
  Constant7 : Constant  Value=3  OutDataTypeStr=fixdt(0, 4, 0)  SampleTime=3.00000003e-08
  From{1..2,4..7,9..12} (10 alike) : hdlmdlgenlib/Buffer
  Goto{1..2,4..8} (7 alike) : hdlmdlgenlib/Buffer
  Logical Operator{,1..5} (6 alike) : Logic  Operator=OR  AllPortsSameDT=off  OutDataTypeStr=boolean  SampleTime=3.00000003e-08
  Multiport Switch : MultiPortSwitch  DataPortForDefault=Additional data port  DiagnosticForDefault=None  OutDataTypeStr=fixdt(1, 33, 15)  SampleTime=3.00000003e-08  SaturateOnIntegerOverflow=off  InputSameDT=off
  Multiport Switch1 : MultiPortSwitch  DataPortForDefault=Additional data port  DiagnosticForDefault=None  OutDataTypeStr=fixdt(1, 33, 15)  SampleTime=3.00000003e-08  SaturateOnIntegerOverflow=off  InputSameDT=off
  Relational Operator : RelationalOperator  Operator=>  OutDataTypeStr=boolean  SampleTime=3.00000003e-08  InputSameDT=off
  Relational Operator{4..14} (11 alike) : RelationalOperator  Operator===  OutDataTypeStr=boolean  SampleTime=3.00000003e-08  InputSameDT=off
  Switch{2..7} (6 alike) : Switch  Criteria=u2 > Threshold  Threshold=double(0)  OutDataTypeStr=fixdt(1, 33, 15)  SampleTime=3.00000003e-08  SaturateOnIntegerOverflow=off  InputSameDT=off
  individual1 : Subsystem
  individual2 : Subsystem
  individual3 : Subsystem
  individual4 : Subsystem
  mux{,1..3} (4 alike) : Mux  Inputs=7
  output_selector : Subsystem
  swap_counter : Subsystem
  swap_counter1 : Subsystem
  t : Constant  Value=double(0)  OutDataTypeStr=boolean  SampleTime=3.00000003e-08
  t{1..4} (4 alike) : Demux  Outputs=7
  individual_out : Outport  SampleTime=3.00000003e-08
  sort_done : Outport  Port=2  SampleTime=3.00000003e-08
  elite_individual : Outport  Port=3  SampleTime=3.00000003e-08
  wires:
  chose_input/1 -> Relational Operator14/1, Relational Operator13/1, Relational Operator12/1, Relational Operator11/1
  start_sorting/1 -> Goto6/1
  chose_output/1 -> Goto7/1
  t/1 -> sort_done/1
  Constant14/1 -> Relational Operator14/2
  Constant5/1 -> Relational Operator11/2
  Constant6/1 -> Relational Operator12/2
  Constant7/1 -> Relational Operator13/2
  From7/1 -> output_selector/1(chose_port)
  mux1/1 -> elite_individual/1, output_selector/2(In2), Switch4/1
  mux2/1 -> output_selector/3(In3), Switch6/1, Switch2/1
  mux3/1 -> output_selector/4(In4), Switch7/1, Switch4/3
  mux/1 -> output_selector/5(In5), Switch6/3
  output_selector/1(Out1) -> individual_out/1
  Goto6/1 -> From2/1
  Goto7/1 -> From7/1
  Chart/3(sort_done) -> Chart_term2/1
  individual3/1(score) -> Multiport Switch/4, Multiport Switch1/3, mux3/1
  individual3/2(a2) -> mux3/2
  individual3/3(a3) -> mux3/3
  individual3/4(a4) -> mux3/4
  individual3/5(b2) -> mux3/5
  individual3/6(b3) -> mux3/6
  individual3/7(b4) -> mux3/7
  individual2/1(score) -> Multiport Switch/3, Multiport Switch1/2, Multiport Switch1/5, mux2/1
  individual2/2(a2) -> mux2/2
  individual2/3(a3) -> mux2/3
  individual2/4(a4) -> mux2/4
  individual2/5(b2) -> mux2/5
  individual2/6(b3) -> mux2/6
  individual2/7(b4) -> mux2/7
  individual1/1(score) -> Multiport Switch/2, Multiport Switch/5, mux1/1
  individual1/2(a2) -> mux1/2
  individual1/3(a3) -> mux1/3
  individual1/4(a4) -> mux1/4
  individual1/5(b2) -> mux1/5
  individual1/6(b3) -> mux1/6
  individual1/7(b4) -> mux1/7
  individual4/1(score) -> Multiport Switch1/4, mux/1
  individual4/2(a2) -> mux/2
  individual4/3(a3) -> mux/3
  individual4/4(a4) -> mux/4
  individual4/5(b2) -> mux/5
  individual4/6(b3) -> mux/6
  individual4/7(b4) -> mux/7
  swap_counter/1(Out1) -> Chart/3(swaps_in)
  swap_counter1/1(Out1) -> Chart/1(index), Multiport Switch/1, Multiport Switch1/1
  Relational Operator13/1 -> Logical Operator4/2
  Constant12/1 -> Relational Operator9/2
  Constant10/1 -> Relational Operator7/2
  Relational Operator12/1 -> Logical Operator3/2
  Constant11/1 -> Relational Operator8/2
  Constant9/1 -> Relational Operator6/2
  Relational Operator11/1 -> Logical Operator2/2
  Constant4/1 -> Relational Operator4/2
  Relational Operator14/1 -> Logical Operator5/2
  Constant13/1 -> Relational Operator10/2
  individual_in/1 -> Switch7/3, Switch5/3, Switch3/3, Switch2/3
  From2/1 -> Chart/2(start_sort)
  Constant8/1 -> Relational Operator5/2
  Logical Operator4/1 -> individual3/8(enable)
  Logical Operator3/1 -> individual2/8(enable)
  Relational Operator4/1 -> individual1/8(enable)
  Logical Operator5/1 -> individual4/8(enable)
  t1/1 -> individual4/1(reg_in)
  t1/2 -> individual4/2(reg_in1)
  t1/3 -> individual4/3(reg_in2)
  t1/4 -> individual4/4(reg_in3)
  t1/5 -> individual4/5(reg_in4)
  t1/6 -> individual4/6(reg_in5)
  t1/7 -> individual4/7(reg_in6)
  From10/1 -> swap_counter/2(In2)
  From9/1 -> swap_counter/1(In1)
  From11/1 -> swap_counter1/2(In2)
  From12/1 -> swap_counter1/1(In1)
  t2/1 -> individual1/1(reg_in)
  t2/2 -> individual1/2(reg_in1)
  t2/3 -> individual1/3(reg_in2)
  t2/4 -> individual1/4(reg_in3)
  t2/5 -> individual1/5(reg_in4)
  t2/6 -> individual1/6(reg_in5)
  t2/7 -> individual1/7(reg_in6)
  t3/1 -> individual2/1(reg_in)
  t3/2 -> individual2/2(reg_in1)
  t3/3 -> individual2/3(reg_in2)
  t3/4 -> individual2/4(reg_in3)
  t3/5 -> individual2/5(reg_in4)
  t3/6 -> individual2/6(reg_in5)
  t3/7 -> individual2/7(reg_in6)
  t4/1 -> individual3/1(reg_in)
  t4/2 -> individual3/2(reg_in1)
  t4/3 -> individual3/3(reg_in2)
  t4/4 -> individual3/4(reg_in3)
  t4/5 -> individual3/5(reg_in4)
  t4/6 -> individual3/6(reg_in5)
  t4/7 -> individual3/7(reg_in6)
  Relational Operator9/1 -> Logical Operator1/2
  Logical Operator1/1 -> Switch5/2, Logical Operator4/1
  From5/1 -> Relational Operator9/1, Relational Operator7/1
  Relational Operator7/1 -> Switch6/2, Logical Operator1/1
  Relational Operator8/1 -> Logical Operator/2
  Logical Operator/1 -> Switch3/2, Logical Operator3/1
  From4/1 -> Relational Operator8/1, Relational Operator6/1
  Relational Operator6/1 -> Switch4/2, Logical Operator/1
  Logical Operator2/1 -> Relational Operator4/1
  From6/1 -> Relational Operator10/1
  Relational Operator10/1 -> Switch7/2, Logical Operator5/1
  Switch7/1 -> t1/1
  Multiport Switch1/1 -> Relational Operator/2
  Multiport Switch/1 -> Relational Operator/1
  Relational Operator/1 -> Chart/4(swap_signal)
  Goto5/1 -> From10/1
  Goto4/1 -> From9/1
  Goto8/1 -> From11/1
  Goto2/1 -> From12/1
  Chart/1(index_increment) -> Goto2/1
  Chart/2(index_reset) -> Goto8/1
  Chart/4(commit_swap) -> Goto1/1
  Chart/5(swaps_increment) -> Goto4/1
  Chart/6(reset_swaps) -> Goto5/1
  Goto1/1 -> From6/1, From5/1, From4/1, From1/1
  From1/1 -> Relational Operator5/1
  Relational Operator5/1 -> Switch2/2, Logical Operator2/1
  Switch2/1 -> t2/1
  Switch4/1 -> Switch3/1
  Switch3/1 -> t3/1
  Switch6/1 -> Switch5/1
  Switch5/1 -> t4/1

== system gm_DUALportRAMinterface_v3/PL/integration_block1/GA_main/generation_counter ==
  In1 : Inport  OutDataTypeStr=boolean  PortDimensions=1  SampleTime=3.00000003e-08
  In2 : Inport  Port=2  OutDataTypeStr=boolean  PortDimensions=1  SampleTime=3.00000003e-08
  Add : Sum  OutDataTypeStr=fixdt(0,16,0)  AccumDataTypeStr=fixdt(0,16,0)
  Constant18 : Constant  OutDataTypeStr=fixdt(0,16,0)  SampleTime=Ts
  Constant19 : Constant  Value=0  OutDataTypeStr=fixdt(0,16,0)  SampleTime=Ts
  Constant20 : Constant  Value=0  OutDataTypeStr=fixdt(0,16,0)  SampleTime=Ts
  Delay : Delay  DelayLength=1  InitialCondition=0  SampleTime=Ts
  Switch : Switch  Criteria=u2 > Threshold  OutDataTypeStr=fixdt(0,16,0)  SaturateOnIntegerOverflow=off  InputSameDT=off
  Switch8 : Switch  Criteria=u2 > Threshold  OutDataTypeStr=fixdt(0,16,0)  SaturateOnIntegerOverflow=off  InputSameDT=off
  Out1 : Outport  SampleTime=3.00000003e-08
  wires:
  In1/1 -> Switch/2
  Constant18/1 -> Switch/1
  Constant19/1 -> Switch/3
  Delay/1 -> Out1/1, Switch8/3
  Constant20/1 -> Switch8/1
  In2/1 -> Switch8/2
  Switch/1 -> Add/1
  Add/1 -> Delay/1
  Switch8/1 -> Add/2
